simulink subsystem "Imu_Publisher"  (R2022a)
settings: Solver=VariableStepAuto  StartTime=0.0  StopTime=10.0  RelTol=1e-3
undefined symbols (not defined in the file or in its folder): angular_velocity, linear_acceleration, orientation
libraries: ros2lib x2
settings Model: Creator=hayden  LastModifiedBy=hollis

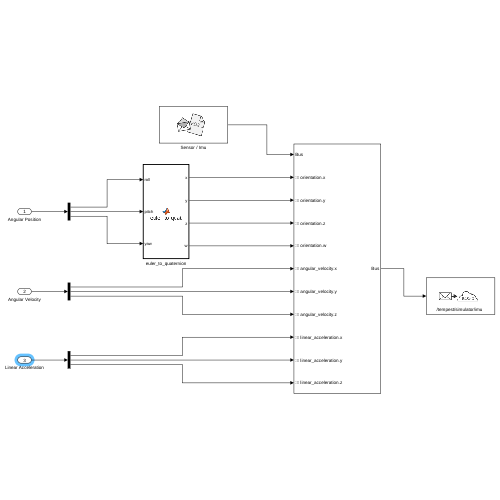
[thumbnail: Simulink's stored preview of the top-level diagram]
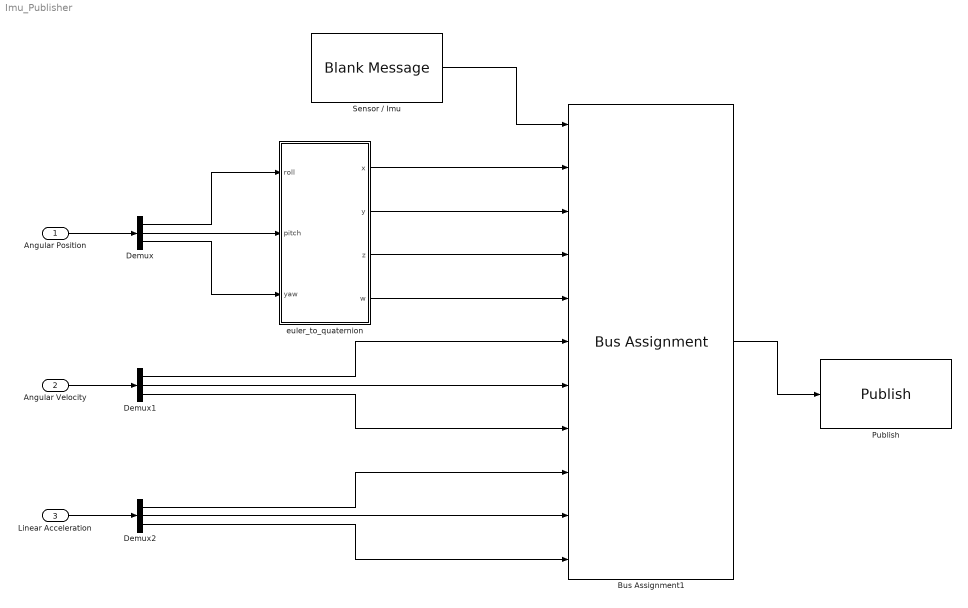
== system Imu_Publisher ==
  Angular Position : Inport
  Angular Velocity : Inport  Port=2
  Linear Acceleration : Inport  Port=3
  Bus Assignment1 : BusAssignment  AssignedSignals=orientation.x,orientation.y,orientation.z,orientation.w,angular_velocity.x,angular_velocity.y,angular_velocity.z,linear_acceleration.x,linear_acceleration.y,linear_acceleration.z
  Demux : Demux  Outputs=3
  Demux1 : Demux  Outputs=3
  Demux2 : Demux  Outputs=3
  Publish : ros2lib/Publish  topicSource=Specify your own  topic=/tempest/simulator/imu  messageType=sensor_msgs/Imu  QOSHistory=Keep last  QOSDepth=1  QOSReliability=Reliable  QOSDurability=Volatile
      settings: SourceProductBaseCode=RR
  Sensor / Imu : ros2lib/Blank Message  messageClass=Message  entityType=sensor_msgs/Imu  messageType=geometry_msgs/Pose  SampleTime=inf
      settings: SourceProductBaseCode=RR
  euler_to_quaternion : MATLAB Function  TreatAsAtomicUnit=on
  wires:
  Sensor / Imu/1 -> Bus Assignment1/1
  euler_to_quaternion/1(x) -> Bus Assignment1/2
  euler_to_quaternion/2(y) -> Bus Assignment1/3
  euler_to_quaternion/3(z) -> Bus Assignment1/4
  euler_to_quaternion/4(w) -> Bus Assignment1/5
  Bus Assignment1/1 -> Publish/1
  Demux/2 -> euler_to_quaternion/2(pitch)
  Demux/1 -> euler_to_quaternion/1(roll)
  Demux/3 -> euler_to_quaternion/3(yaw)
  Demux1/2 -> Bus Assignment1/7
  Demux1/1 -> Bus Assignment1/6
  Demux1/3 -> Bus Assignment1/8
  Demux2/2 -> Bus Assignment1/10
  Demux2/1 -> Bus Assignment1/9
  Demux2/3 -> Bus Assignment1/11
  Angular Position/1 -> Demux/1
  Linear Acceleration/1 -> Demux2/1
  Angular Velocity/1 -> Demux1/1

== matlab function Imu_Publisher/euler_to_quaternion ==
  data: roll input; x output; pitch input; yaw input; y output; z output; w output
function [x,y,z,w]= euler_to_quat(roll, pitch, yaw)
    euler = [roll, pitch, yaw];
    SEQ = "XYZ";
    quat = eul2quat(euler, SEQ);
    x = quat(1);
    y = quat(2);
    z = quat(3);
    w = quat(4);
